simulink model "mod2_SS_2bit"  (R2013a)
settings: Solver=FixedStepDiscrete  StartTime=0.0  StopTime=80e-3  RelTol=1e-3
undefined symbols (not defined in the file): Fs, modctrl
libraries: dspsigops x2, dspsrcs4 x1
settings Model: Creator=amyles  LastModifiedBy=amyles
settings DataIOCC: LimitDataPoints=off  MaxDataPoints=50000  SignalLoggingSaveFormat=ModelDataLogs
settings OptimizationCC: InlineParams=on  ExpressionDepthLimit=2147483647
settings DebuggingCC: FcnCallInpInsideContextMsg=UseLocalSettings  StrictBusMsg=Warning
settings ModelReferenceCC: ModelReferenceNumInstancesAllowed=Single
settings GRTTargetCC: CombineOutputUpdateFcns=off  GRTInterface=on

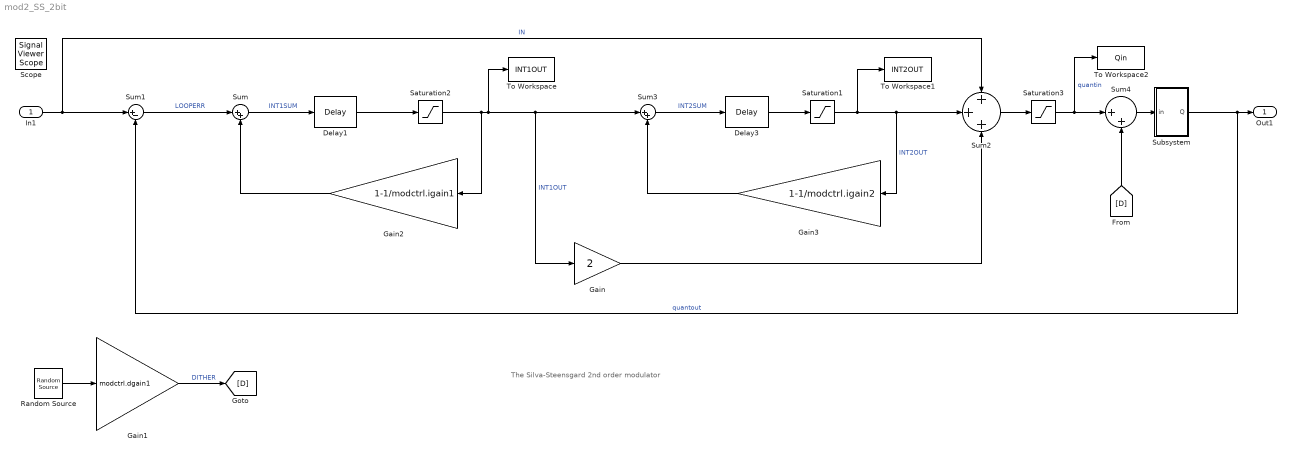
== system mod2_SS_2bit ==
  note: The Silva-Steensgard 2nd order modulator
  In1 : Inport
  Delay1 : dspsigops/Delay  InputProcessing=Inherited (this choice will be removed - see release notes)  dly_unit=Samples  delay=1  ic_detail=off  dif_ic_for_ch=off  dif_ic_for_dly=off  ic=0.05  reset_popup=None
  Delay3 : dspsigops/Delay  InputProcessing=Inherited (this choice will be removed - see release notes)  dly_unit=Samples  delay=1  ic_detail=off  dif_ic_for_ch=off  dif_ic_for_dly=off  ic=0.05  reset_popup=None
  Gain : Gain  Gain=2
  Gain1 : Gain  Gain=modctrl.dgain1
      settings: AttributesFormatString=Dither level adjust
  Gain2 : Gain  Gain=1-1/modctrl.igain1
      settings: AttributesFormatString=Integrator leakage
  Gain3 : Gain  Gain=1-1/modctrl.igain2
      settings: AttributesFormatString=Integrator leakage
  Random Source : dspsrcs4/Random Source  SrcType=Uniform  NormMethod=Ziggurat  CltLength=12  MinVal=-1  MaxVal=1  MeanVal=0  VarVal=1  RepMode=Not repeatable  rawSeed=1  IsInherit=off  SampMode=Discrete  SampTime=1/Fs  SampFrame=1  DataType=Double  OutComplex=Real
      settings: AttributesFormatString=Dither source
  Saturation1 : Saturate  UpperLimit=modctrl.isat2  LowerLimit=-(modctrl.isat2)
  Saturation2 : Saturate  UpperLimit=modctrl.isat1  LowerLimit=-(modctrl.isat1)
  Saturation3 : Saturate  UpperLimit=modctrl.qsatin1  LowerLimit=-(modctrl.qsatin1)
  Subsystem : Subsystem
      settings: AttributesFormatString=2-bit quantiser
  Sum : Sum  Inputs=|++
      settings: AttributesFormatString=Integrator summer
  Sum1 : Sum  Inputs=|+-
      settings: AttributesFormatString=Modulator input\nloop servo error (input - fbk)
  Sum2 : Sum  Inputs=+++
  Sum3 : Sum  Inputs=|++
      settings: AttributesFormatString=Integrator summer
  Sum4 : Sum  Inputs=|++
  To Workspace : ToWorkspace  VariableName=INT1OUT  SampleTime=-1
  To Workspace1 : ToWorkspace  VariableName=INT2OUT  SampleTime=-1
  To Workspace2 : ToWorkspace  VariableName=Qin  SampleTime=-1
  Out1 : Outport
  Scope : SignalViewerScope  IOType=viewer  NumInputPorts=4  ZoomMode=yonly  RefreshTime=0.035000
      settings: YMin=-5~-5~-5~-5  YMax=5~5~5~5
  wires:
  Sum/1 -> Delay1/1  "INT1SUM"
  Sum1/1 -> Sum/1  "LOOPERR"
  In1/1 -> Sum1/1, Sum2/1  "IN"
  Gain2/1 -> Sum/2
  Sum3/1 -> Delay3/1  "INT2SUM"
  Gain3/1 -> Sum3/2
  Saturation1/1 -> Gain3/1, Sum2/2, To Workspace1/1  "INT2OUT"
  Saturation2/1 -> Gain2/1, Sum3/1, Gain/1, To Workspace/1  "INT1OUT"
  Random Source/1 -> Gain1/1
  Delay3/1 -> Saturation1/1
  Delay1/1 -> Saturation2/1
  Gain/1 -> Sum2/3
  Gain1/1 -> [D]  "DITHER"
  Sum2/1 -> Saturation3/1
  Saturation3/1 -> Sum4/1, To Workspace2/1  "quantin"
  Sum4/1 -> Subsystem/1(in)
  [D] -> Sum4/2
  Subsystem/1(Q) -> Out1/1, Sum1/2  "quantout"

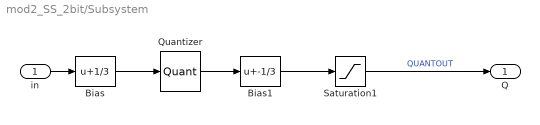
== system mod2_SS_2bit/Subsystem ==
  in : Inport
  Bias : Bias  Bias=1/3
      settings: AttributesFormatString=Need offset to give\nMID-RISE quantiser
  Bias1 : Bias  Bias=-1/3
  Quantizer : Quantizer  QuantizationInterval=2/3  LinearizeAsGain=off
  Saturation1 : Saturate  UpperLimit=1  LowerLimit=-1
      settings: AttributesFormatString=Limit quantiser\noutput to +/-1
  Q : Outport
  wires:
  Saturation1/1 -> Q/1  "QUANTOUT"
  in/1 -> Bias/1
  Bias1/1 -> Saturation1/1
  Quantizer/1 -> Bias1/1
  Bias/1 -> Quantizer/1
